simulink model "Tqs"  (R2021a)
settings: Solver=ode45  StartTime=0.0  StopTime=10.0  RelTol=1e-3  EnableMultiTasking=on
undefined symbols (not defined in the file): Tqs_facKIdleSpdCtrl, Tqs_flgIdleSpdCtrlEnable, Tqs_flgTorqueReqOverride, Tqs_rpmEngSpdIdle, Tqs_tiTnIdleSpdCtrl, Tqs_tiTvIdleSpdCtrl, Tqs_tqIdleSpdCtrlMax, Tqs_tqIdleSpdCtrlMin, Tqs_tqReqMan
libraries: simulink x4
settings Model: Creator=YAL9FE  LastModifiedBy=FPR9FE
settings SolverCC: AlgebraicLoopSolver=TrustRegion
settings DataIOCC: LimitDataPoints=on  SaveFormat=Array  SignalLoggingSaveFormat=ModelDataLogs  ReturnWorkspaceOutputs=off
settings OptimizationCC: ExpressionDepthLimit=2147483647  LifeSpan=inf
settings DebuggingCC: UnderspecifiedInitializationDetection=Classic  MergeDetectMultiDrivingBlocksExec=none  SolverPrmCheckMsg=warning  FcnCallInpInsideContextMsg=warning  StateNameClashWarn=warning  SFUnexpectedBacktrackingDiag=warning  SFNoUnconditionalDefaultTransitionDiag=warning  SFExecutionAtInitializationDiag=none  SFMachineParentedDataDiag=warning  ArithmeticOperatorsInVariantConditions=warning
settings HardwareCC: ProdBitPerPointer=32  ProdBitPerSizeT=32  ProdBitPerPtrDiffT=32  ProdLargestAtomicFloat=None  ProdIntDivRoundTo=Undefined  ProdEndianess=Unspecified  ProdWordSize=32  ProdHWDeviceType=32-bit Generic
settings ModelReferenceCC: PropagateSignalLabelsOutOfModel=off
settings SFSimCC: SimUseLocalCustomCode=off  CustomCodeUndefinedFunction=UseInterfaceOnly
settings RTWCC: RTWUseLocalCustomCode=off
settings CodeAppCC: StateflowObjectComments=on
settings GRTTargetCC: TargetLangStandard=C89/C90 (ANSI)  CombineOutputUpdateFcns=off  GRTInterface=on
settings ConfigComp: CovMetricSettings=dw  CovSaveCumulativeToWorkspaceVar=on  CovSaveSingleToWorkspaceVar=on  CovExternalEMLEnable=off  CovSFcnEnable=off

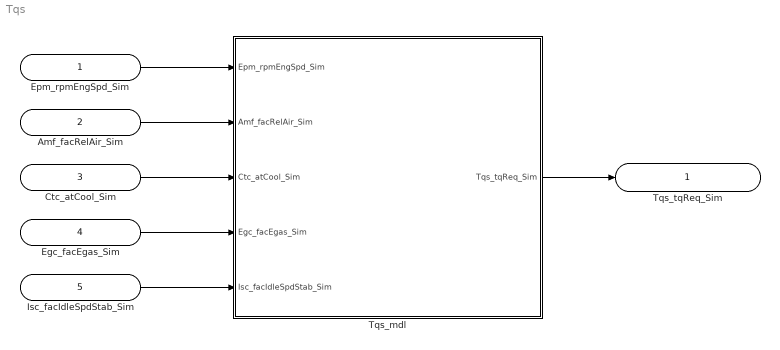
== system Tqs ==
  Epm_rpmEngSpd_Sim : Inport
  Amf_facRelAir_Sim : Inport  Port=2
  Ctc_atCool_Sim : Inport  Port=3
  Egc_facEgas_Sim : Inport  Port=4
  Isc_facIdleSpdStab_Sim : Inport  Port=5
  Tqs_mdl : Subsystem  mask(Functions){}
      mask help: TorqueStructure
      mask Display:
      | image(imread('TorqueStructure.jpg'))
      | port_label('input',1,'Epm_rpmEngSpd_Sim')
      | port_label('input',2,'Amf_facRelAir_Sim')
      | port_label('input',3,'Ctc_atCool_Sim')
      | port_label('input',4,'Egc_facEgas_Sim')
      | port_label('input',5,'Isc_facIdleSpdStab_Sim')
      | port_label('output',1,'Tqs_tqReq_Sim')
  Tqs_tqReq_Sim : Outport
  wires:
  Epm_rpmEngSpd_Sim/1 -> Tqs_mdl/1(Epm_rpmEngSpd_Sim)
  Amf_facRelAir_Sim/1 -> Tqs_mdl/2(Amf_facRelAir_Sim)
  Ctc_atCool_Sim/1 -> Tqs_mdl/3(Ctc_atCool_Sim)
  Egc_facEgas_Sim/1 -> Tqs_mdl/4(Egc_facEgas_Sim)
  Isc_facIdleSpdStab_Sim/1 -> Tqs_mdl/5(Isc_facIdleSpdStab_Sim)
  Tqs_mdl/1(Tqs_tqReq_Sim) -> Tqs_tqReq_Sim/1

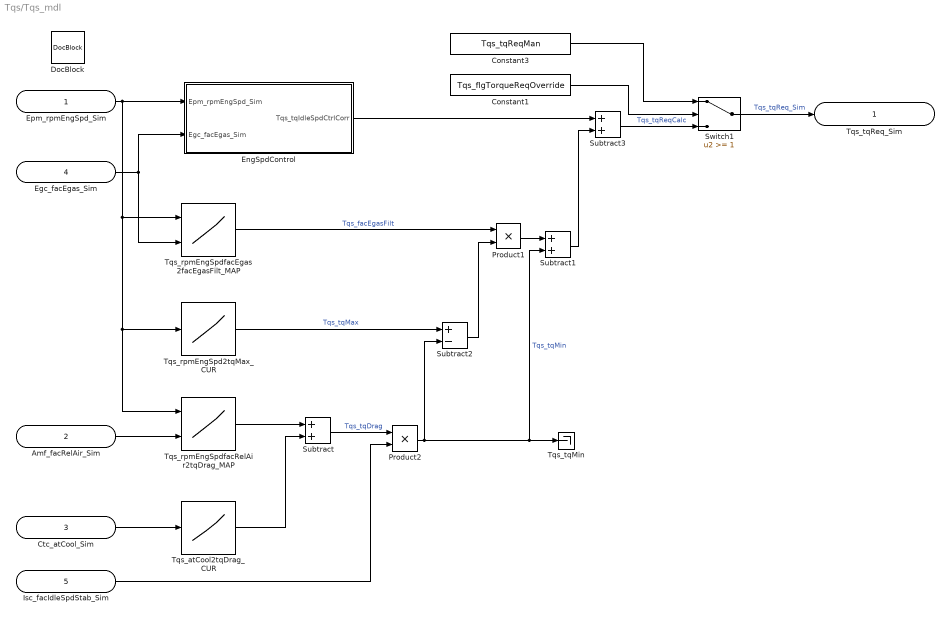
== system Tqs/Tqs_mdl ==
  Epm_rpmEngSpd_Sim : Inport
  Amf_facRelAir_Sim : Inport  Port=2
  Ctc_atCool_Sim : Inport  Port=3
  Egc_facEgas_Sim : Inport  Port=4
  Isc_facIdleSpdStab_Sim : Inport  Port=5
  Constant1 : Constant  Value=Tqs_flgTorqueReqOverride
  Constant3 : Constant  Value=Tqs_tqReqMan
  DocBlock : simulink/Model-Wide Utilities/DocBlock  DocumentType=Text
      content=|
      | The torque structure module (TorqueStructure) calculates the required torque that the engine must provide in order to keep itself running and to meet the driver's request. For self-preservation, the motor must deliver as much torque as is consumed by internal losses (drag torque Tqs_tqDrag ). It is estimated as a function of the speed Epm_rpmEngSpd_Sim and the relative filling Amf_facRelAir_Sim using the map Tqs_rpmEngSpdfacRelAir2tqDrag_MAP. Basically, one can say that at high speeds there is more friction, which leads to greater drag torque, than at low speeds. In addition, there is a correction by the coolant temperature Ctc_atCool_Sim via the map Tqs_atCool2tqDrag_CUR . At very low temperatures, the drag torque increases due to the high viscosity of the engine oil. From a temperature of around 60 degrees Celsius it becomes zero.
  EngSpdControl : Subsystem
  Product1 : Product  OutDataTypeStr=Inherit: Same as first input
  Product2 : Product  OutDataTypeStr=Inherit: Same as first input
  Subtract : Sum  OutDataTypeStr=Inherit: Same as first input
  Subtract1 : Sum  OutDataTypeStr=Inherit: Same as first input
  Subtract2 : Sum  Inputs=+-  OutDataTypeStr=Inherit: Same as first input
  Subtract3 : Sum  OutDataTypeStr=Inherit: Same as first input
  Switch1 : Switch  Threshold=1
  Tqs_atCool2tqDrag_CUR : Lookup_n-D  NumberOfTableDimensions=1  BreakpointsForDimension1=[1:3]  Table=[1 4 9]  ExtrapMethod=Clip  InputSameDT=on
  Tqs_rpmEngSpd2tqMax_CUR : Lookup_n-D  NumberOfTableDimensions=1  BreakpointsForDimension1=[1:3]  Table=[1 4 9]  ExtrapMethod=Clip  InputSameDT=on
  Tqs_rpmEngSpdfacEgas2facEgasFilt_MAP : Lookup_n-D  BreakpointsForDimension1=[1:3]  BreakpointsForDimension2=[1:3]  ExtrapMethod=Clip  InputSameDT=on
      settings: InputPortMap=u0,u1
  Tqs_rpmEngSpdfacRelAir2tqDrag_MAP : Lookup_n-D  BreakpointsForDimension1=[1:3]  BreakpointsForDimension2=[1:3]  ExtrapMethod=Clip  InputSameDT=on
      settings: InputPortMap=u0,u1
  Tqs_tqMin : Terminator
  Tqs_tqReq_Sim : Outport
  wires:
  Constant3/1 -> Switch1/1
  Constant1/1 -> Switch1/2
  Epm_rpmEngSpd_Sim/1 -> EngSpdControl/1(Epm_rpmEngSpd_Sim), Tqs_rpmEngSpd2tqMax_CUR/1, Tqs_rpmEngSpdfacRelAir2tqDrag_MAP/1, Tqs_rpmEngSpdfacEgas2facEgasFilt_MAP/1
  Egc_facEgas_Sim/1 -> EngSpdControl/2(Egc_facEgas_Sim), Tqs_rpmEngSpdfacEgas2facEgasFilt_MAP/2
  Amf_facRelAir_Sim/1 -> Tqs_rpmEngSpdfacRelAir2tqDrag_MAP/2
  Ctc_atCool_Sim/1 -> Tqs_atCool2tqDrag_CUR/1
  Tqs_rpmEngSpdfacRelAir2tqDrag_MAP/1 -> Subtract/1
  Tqs_atCool2tqDrag_CUR/1 -> Subtract/2
  Switch1/1 -> Tqs_tqReq_Sim/1  "Tqs_tqReq_Sim"
  Tqs_rpmEngSpdfacEgas2facEgasFilt_MAP/1 -> Product1/1  "Tqs_facEgasFilt"
  Subtract2/1 -> Product1/2
  Tqs_rpmEngSpd2tqMax_CUR/1 -> Subtract2/1  "Tqs_tqMax"
  Product1/1 -> Subtract1/1
  Product2/1 -> Subtract1/2, Tqs_tqMin/1, Subtract2/2  "Tqs_tqMin"
  Subtract/1 -> Product2/1  "Tqs_tqDrag"
  Isc_facIdleSpdStab_Sim/1 -> Product2/2
  EngSpdControl/1(Tqs_tqIdleSpdCtrlCorr) -> Subtract3/1
  Subtract1/1 -> Subtract3/2
  Subtract3/1 -> Switch1/3  "Tqs_tqReqCalc"

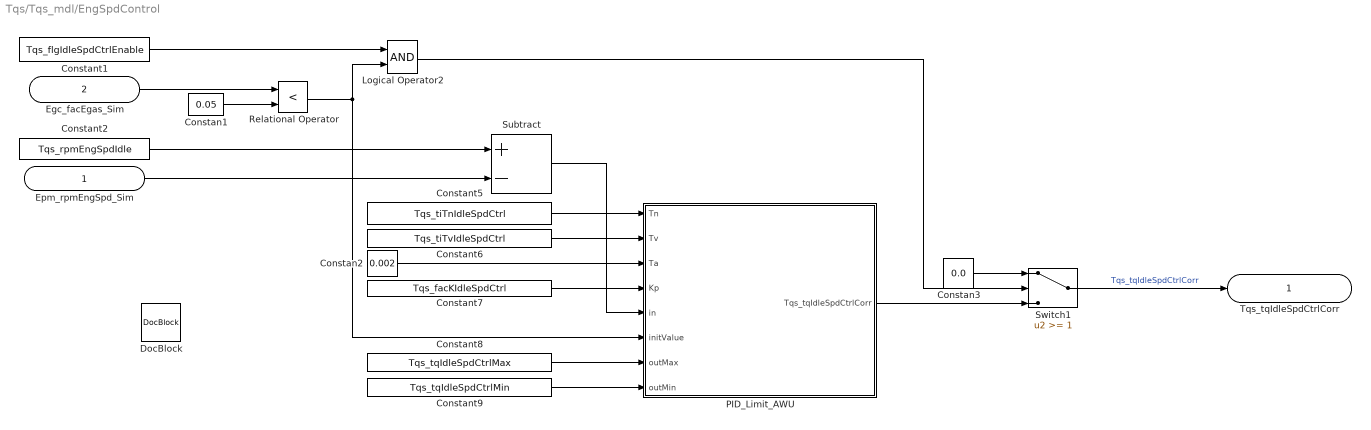
== system Tqs/Tqs_mdl/EngSpdControl ==
  Epm_rpmEngSpd_Sim : Inport
  Egc_facEgas_Sim : Inport  Port=2
  Constan1 : Constant  Value=0.05  OutDataTypeStr=single
  Constan2 : Constant  Value=0.002  OutDataTypeStr=single
  Constan3 : Constant  Value=0.0  OutDataTypeStr=single
  Constant1 : Constant  Value=Tqs_flgIdleSpdCtrlEnable
  Constant2 : Constant  Value=Tqs_rpmEngSpdIdle
  Constant5 : Constant  Value=Tqs_tiTnIdleSpdCtrl
  Constant6 : Constant  Value=Tqs_tiTvIdleSpdCtrl
  Constant7 : Constant  Value=Tqs_facKIdleSpdCtrl
  Constant8 : Constant  Value=Tqs_tqIdleSpdCtrlMax
  Constant9 : Constant  Value=Tqs_tqIdleSpdCtrlMin
  DocBlock : simulink/Model-Wide Utilities/DocBlock  DocumentType=Text
      content=|
      | The engine should maintain a stable idling speed without the driver requesting it, i. i.e. the torque requirement must correspond to the drag torque. At high engine speeds, the torque request should decrease without the driver's desired torque so that the engine speed is reduced (engine braking) and increase at lower engine speeds than the idling speed so that the engine does not stall. This is achieved by calculating a speed-dependent minimum torque. To do this, the stabilization factor Tqs_facEngSpdStab is calculated by dividing the idle speed Tqs_rpmTorqueInc and the current speed and multiplied by the drag torque. At high speeds, the minimum required torque is less than the drag torque, so the engine brakes. At idle speed, the factor becomes one, i. This means that the drag torque is exactly balanced and at speeds below idle speed there is an overshoot, so that the engine accelerates and tries to reach idle speed. Forming the maximum of speed and one serves to prevent division by zero under all circumstances.
  Logical Operator2 : Logic  AllPortsSameDT=off  OutDataTypeStr=boolean
  PID_Limit_AWU : Subsystem
      mask help: PID_Limit_AWU
      mask Display:
      | image(imread('PID_Limit_AWU.jpg'))
      | port_label('input',1,'Tn')
      | port_label('input',2,'Tv')
      | port_label('input',3,'Ta')
      | port_label('input',4,'Kp')
      | port_label('input',5,'in')
      | port_label('input',6,'initValue')
      | port_label('input',7,'outMax')
      | port_label('input',8,'outMin')
      | port_label('output',1,'Tqs_tqIdleSpdCtrlCorr')
  Relational Operator : RelationalOperator  Operator=<  OutDataTypeStr=boolean  RndMeth=Nearest
  Subtract : Sum  Inputs=+-  OutDataTypeStr=Inherit: Same as first input
  Switch1 : Switch  Threshold=1
  Tqs_tqIdleSpdCtrlCorr : Outport
  wires:
  PID_Limit_AWU/1(Tqs_tqIdleSpdCtrlCorr) -> Switch1/3
  Constan1/1 -> Relational Operator/2
  Switch1/1 -> Tqs_tqIdleSpdCtrlCorr/1  "Tqs_tqIdleSpdCtrlCorr"
  Constant5/1 -> PID_Limit_AWU/1(Tn)
  Constan2/1 -> PID_Limit_AWU/3(Ta)
  Subtract/1 -> PID_Limit_AWU/5(in)
  Constant6/1 -> PID_Limit_AWU/2(Tv)
  Constant7/1 -> PID_Limit_AWU/4(Kp)
  Epm_rpmEngSpd_Sim/1 -> Subtract/2
  Constant2/1 -> Subtract/1
  Constant8/1 -> PID_Limit_AWU/7(outMax)
  Constant9/1 -> PID_Limit_AWU/8(outMin)
  Constan3/1 -> Switch1/1
  Constant1/1 -> Logical Operator2/1
  Relational Operator/1 -> Logical Operator2/2, PID_Limit_AWU/6(initValue)
  Egc_facEgas_Sim/1 -> Relational Operator/1
  Logical Operator2/1 -> Switch1/2

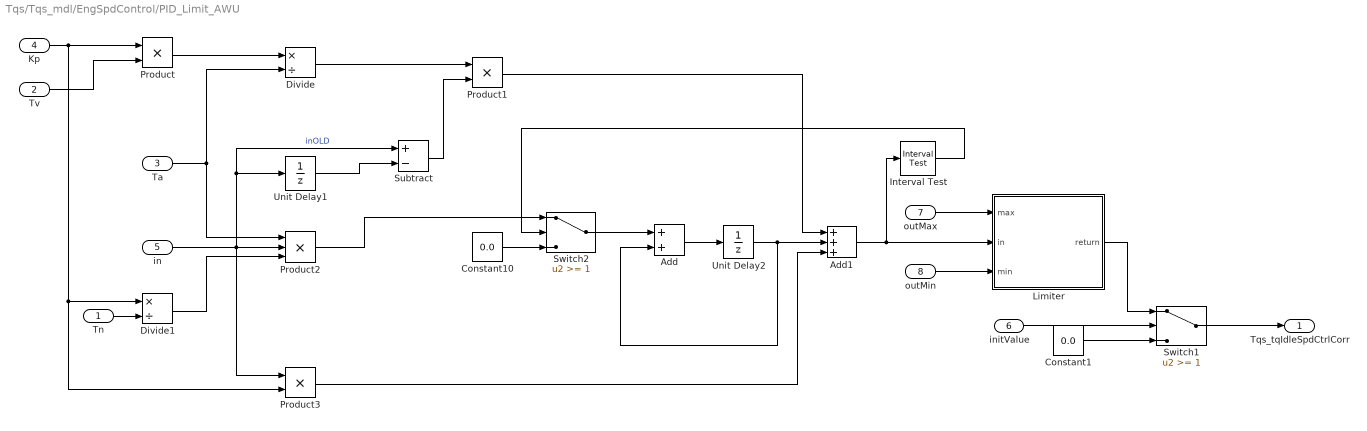
== system Tqs/Tqs_mdl/EngSpdControl/PID_Limit_AWU ==
  Tn : Inport
  Tv : Inport  Port=2
  Ta : Inport  Port=3
  Kp : Inport  Port=4
  in : Inport  Port=5
  initValue : Inport  Port=6
  outMax : Inport  Port=7
  outMin : Inport  Port=8
  Add : Sum  OutDataTypeStr=Inherit: Same as first input
  Add1 : Sum  Inputs=+++  OutDataTypeStr=Inherit: Same as first input
  Constant1 : Constant  Value=0.0  OutDataTypeStr=single
  Constant10 : Constant  Value=0.0  OutDataTypeStr=single
  Divide : Product  Inputs=*/  OutDataTypeStr=Inherit: Same as first input
  Divide1 : Product  Inputs=*/  OutDataTypeStr=Inherit: Same as first input
  Interval Test : simulink/Logic and Bit Operations/Interval Test  IntervalClosedRight=on  uplimit=Tqs_tqIdleSpdCtrlMax  IntervalClosedLeft=on  lowlimit=Tqs_tqIdleSpdCtrlMin  OutDataTypeStr=boolean
  Limiter : Subsystem
      mask help: Limiter
      mask Display: image(imread('Limiter.jpg'))
  Product : Product  OutDataTypeStr=Inherit: Same as first input
  Product1 : Product  OutDataTypeStr=Inherit: Same as first input
  Product2 : Product  Inputs=3  OutDataTypeStr=Inherit: Same as first input
  Product3 : Product  OutDataTypeStr=Inherit: Same as first input
  Subtract : Sum  Inputs=+-  OutDataTypeStr=Inherit: Same as first input
  Switch1 : Switch  Threshold=1
  Switch2 : Switch  Threshold=1
  Unit Delay1 : UnitDelay  SampleTime=-1  HasFrameUpgradeWarning=on
  Unit Delay2 : UnitDelay  SampleTime=-1  HasFrameUpgradeWarning=on
  Tqs_tqIdleSpdCtrlCorr : Outport
  wires:
  Constant10/1 -> Switch2/3
  Product2/1 -> Switch2/1
  Interval Test/1 -> Switch2/2
  Unit Delay2/1 -> Add/2, Add1/2
  Add/1 -> Unit Delay2/1
  Unit Delay1/1 -> Subtract/2
  Kp/1 -> Product/1, Product3/2, Divide1/1
  Tv/1 -> Product/2
  Product/1 -> Divide/1
  Ta/1 -> Product2/1, Divide/2
  Divide/1 -> Product1/1
  Tn/1 -> Divide1/2
  in/1 -> Product2/2, Product3/1, Subtract/1, Unit Delay1/1  "inOLD"
  Divide1/1 -> Product2/3
  Subtract/1 -> Product1/2
  Switch2/1 -> Add/1
  Product3/1 -> Add1/3
  Product1/1 -> Add1/1
  Add1/1 -> Limiter/2(in), Interval Test/1
  outMin/1 -> Limiter/3(min)
  outMax/1 -> Limiter/1(max)
  Constant1/1 -> Switch1/3
  initValue/1 -> Switch1/2
  Switch1/1 -> Tqs_tqIdleSpdCtrlCorr/1
  Limiter/1(return) -> Switch1/1

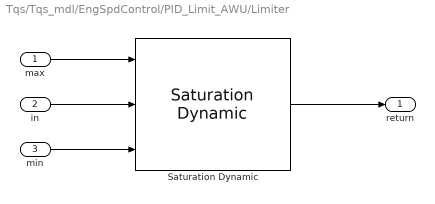
== system Tqs/Tqs_mdl/EngSpdControl/PID_Limit_AWU/Limiter ==
  max : Inport
  in : Inport  Port=2
  min : Inport  Port=3
  Saturation Dynamic : simulink/Discontinuities/Saturation Dynamic  OutMin=[]  OutMax=[]  OutDataTypeStr=Inherit: Same as second input  OutDataType=fixdt(1, 16)  OutScaling=2^-10  DoSatur=off
  return : Outport
  wires:
  max/1 -> Saturation Dynamic/1
  in/1 -> Saturation Dynamic/2
  min/1 -> Saturation Dynamic/3
  Saturation Dynamic/1 -> return/1
